simulink model "PID_controller"  (R2021b)
settings: Solver=VariableStepAuto  StartTime=0.0  StopTime=10.0  RelTol=1e-3
settings Model: Creator=mahima  LastModifiedBy=mahima

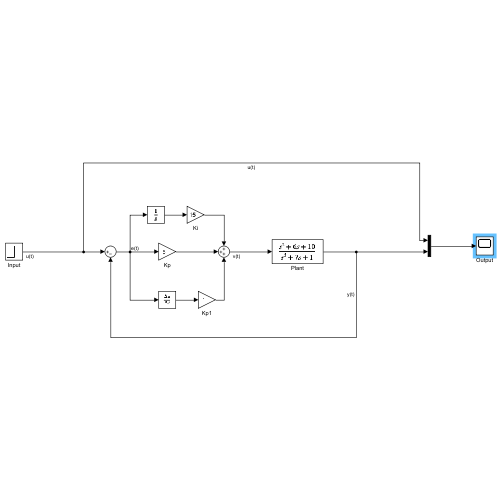
[thumbnail: Simulink's stored preview of the top-level diagram]
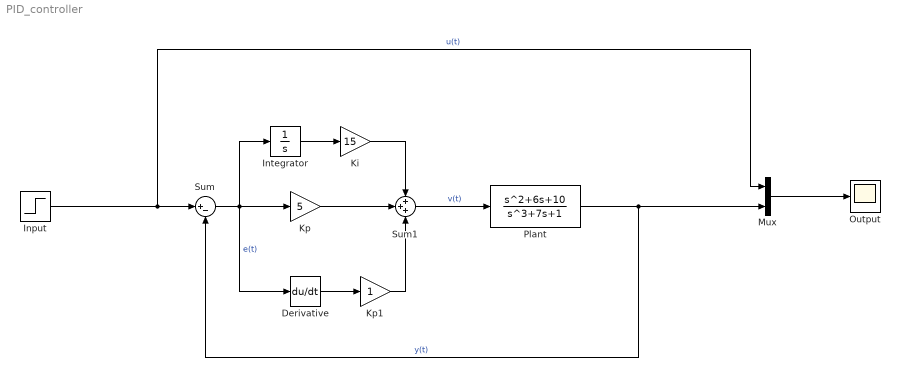
== system PID_controller ==
  Derivative : Derivative
  Input : Step  SampleTime=0
  Integrator : Integrator
  Ki : Gain  Gain=15
  Kp : Gain  Gain=5
  Kp1 : Gain
  Mux : Mux  Inputs=2
  Output : Scope
  Plant : TransferFcn  Numerator=[1,6,10]  Denominator=[1,0,7,1]
  Sum : Sum  Inputs=|+-
  Sum1 : Sum  Inputs=+++
  wires:
  Sum1/1 -> Plant/1  "v(t)"
  Ki/1 -> Sum1/1
  Input/1 -> Mux/1, Sum/1  "u(t)"
  Plant/1 -> Sum/2, Mux/2  "y(t)"
  Sum/1 -> Derivative/1, Integrator/1, Kp/1  "e(t)"
  Mux/1 -> Output/1
  Integrator/1 -> Ki/1
  Kp/1 -> Sum1/2
  Derivative/1 -> Kp1/1
  Kp1/1 -> Sum1/3
